simulink model "LQ_B"  (R2023b)
settings: Solver=ode45  StartTime=0.0  StopTime=80  FixedStep=0.001  MaxStep=.01  RelTol=1e-3  EnableMultiTasking=on
values from neighbouring files (symbols this model uses):
  A = [0 1 0 ... (first row only)    [tf2ss_3rzad.m]
undefined symbols (not defined in the file or in its folder): B, C, h, xo, xo_obs
settings Model: Creator=RGrygiel  LastModifiedBy=pc
settings SolverCC: AlgebraicLoopSolver=TrustRegion
settings DataIOCC: SaveFormat=Array  SignalLoggingSaveFormat=ModelDataLogs  ReturnWorkspaceOutputs=off  SignalLoggingName=sigsOut
settings OptimizationCC: ExpressionDepthLimit=2147483647  InitFltsAndDblsToZero=on  LifeSpan=inf
settings DebuggingCC: SaveWithParameterizedLinksMsg=none  UnderspecifiedInitializationDetection=Classic  MergeDetectMultiDrivingBlocksExec=none  SignalResolutionControl=TryResolveAllWithWarning  MultiTaskDSMMsg=warning  MultiTaskCondExecSysMsg=none  FcnCallInpInsideContextMsg=warning  UnconnectedInputMsg=warning  UnconnectedOutputMsg=warning  UnconnectedLineMsg=warning  StateNameClashWarn=warning  SFUnexpectedBacktrackingDiag=warning  SFNoUnconditionalDefaultTransitionDiag=warning  SFExecutionAtInitializationDiag=none  ArithmeticOperatorsInVariantConditions=warning
settings HardwareCC: ProdBitPerPointer=32  ProdBitPerSizeT=32  ProdBitPerPtrDiffT=32  ProdLargestAtomicFloat=None  ProdIntDivRoundTo=Undefined  ProdEndianess=Unspecified  ProdWordSize=32  ProdHWDeviceType=32-bit Generic  TargetUnknown=on
settings ModelReferenceCC: PropagateSignalLabelsOutOfModel=off
settings CodeAppCC: StateflowObjectComments=on
settings GRTTargetCC: TargetLangStandard=C89/C90 (ANSI)  CombineOutputUpdateFcns=off  GRTInterface=on
settings ConfigComp: CovMetricSettings=dw  CovSaveCumulativeToWorkspaceVar=on  CovSaveSingleToWorkspaceVar=on

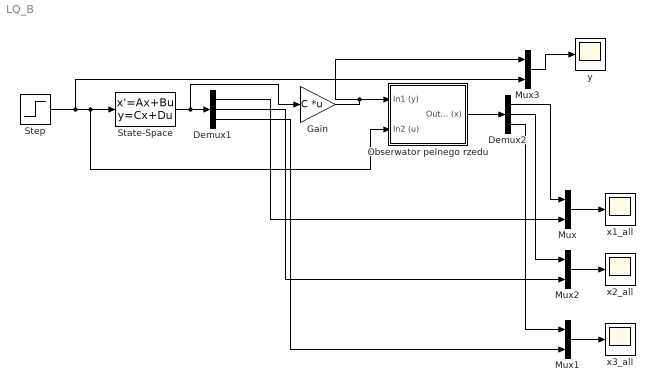
== system LQ_B ==
  Demux1 : Demux  Outputs=3
      settings: DisplayOption=none
  Demux2 : Demux  Outputs=3
      settings: DisplayOption=none
  Gain : Gain  Gain=C  Multiplication=Matrix(K*u) (u vector)  SaturateOnIntegerOverflow=on  OutDataTypeStr=Inherit: Same as input  ParamDataTypeStr=Inherit: Same as input
  Mux{,1..3} (4 alike) : Mux  Inputs=2
  Obserwator pelnego rzedu : Subsystem  mask{H=h, xo_obs=xo_obs}
      mask prompts: xo_obs "war. poczakowy x(0)"
  State-Space : StateSpace  A=A  B=B  C=C  D=zeros(3,1)  InitialCondition=xo
  Step : Step  Time=40  After=10  SampleTime=0
  x1_all : Scope
  x2_all : Scope
  x3_all : Scope
  y : Scope
  wires:
  Step/1 -> State-Space/1, Obserwator pelnego rzedu/2(In2 (u)), Mux3/2
  State-Space/1 -> Demux1/1, Gain/1
  Mux/1 -> x1_all/1
  Mux2/1 -> x2_all/1
  Mux1/1 -> x3_all/1
  Demux2/2 -> Mux2/1
  Demux2/3 -> Mux1/1
  Obserwator pelnego rzedu/1(Out1 (x)) -> Demux2/1
  Demux2/1 -> Mux/1
  Mux3/1 -> y/1
  Gain/1 -> Mux3/1, Obserwator pelnego rzedu/1(In1 (y))
  Demux1/1 -> Mux/2
  Demux1/2 -> Mux2/2
  Demux1/3 -> Mux1/2

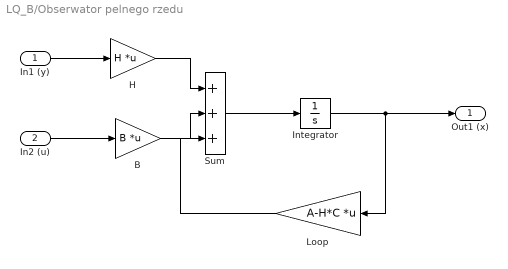
== system LQ_B/Obserwator pelnego rzedu ==
  In1 (y) : Inport
  In2 (u) : Inport  Port=2
  B : Gain  Gain=B  Multiplication=Matrix(K*u) (u vector)  SaturateOnIntegerOverflow=on  OutDataTypeStr=Inherit: Same as input  ParamDataTypeStr=Inherit: Same as input
  H : Gain  Gain=H  Multiplication=Matrix(K*u) (u vector)  SaturateOnIntegerOverflow=on  OutDataTypeStr=Inherit: Same as input  ParamDataTypeStr=Inherit: Same as input
  Integrator : Integrator  InitialCondition=xo_obs
  Loop : Gain  Gain=A-H*C  Multiplication=Matrix(K*u) (u vector)  SaturateOnIntegerOverflow=on  OutDataTypeStr=Inherit: Same as input  ParamDataTypeStr=Inherit: Same as input
  Sum : Sum  Inputs=|+++  SaturateOnIntegerOverflow=on
  Out1 (x) : Outport
  wires:
  Sum/1 -> Integrator/1
  Integrator/1 -> Loop/1, Out1 (x)/1
  Loop/1 -> Sum/3
  B/1 -> Sum/2
  H/1 -> Sum/1
  In1 (y)/1 -> H/1
  In2 (u)/1 -> B/1
